simulink model "motor_dc_simulink"  (R2020a)
settings: Solver=VariableStepAuto  StartTime=0.0  StopTime=60  RelTol=1e-3
values from neighbouring files (symbols this model uses):
  b = 0    [Ex_AproximacaoDiscreta.m]    (also in Ex_PeriodoDeAmostragem1.m = 10; Ex_PeriodoDeAmostragem2.m = 17; motor_dc.m = 0.1)
  J = 0.01    [motor_dc.m]
  K = [0:0.001:30]    [Ex_LugarDasRaizes.m]    (also in Ex_ProjetoCtrlDireto.m = [0:0.005:50]; Ex_ProjetoCtrlDireto2.m = [0:0.001:50]; Ex_ProjetoCtrlEmulacao.m = [0:0.001:20]; Ex_ProjetoObsOrdemReduzida.m = [zeros(1,size(A,1)-1)  1]*inv(Co)*( A^2 + alphaccz(2)*A + al)
  L = [l1 l2]'    [Ex_ProjetoObservador.m]    (also in Ex_ProjetoObservador2.m = ( A^2 + alphacz(2)*A + alphacz(3)*eye(size(A)) )*inv(Ob)*[ze; Ex_ProjetoRastreamento.m = ( A^2 + alphacz(2)*A + alphacz(3)*eye(size(A)) )*inv(Ob)*[ze; motor_dc.m = 0.5)
  R = 1    [motor_dc.m]
  T = 0.1    [Ex_AproximacaoDiscreta.m]    (also in Ex_DiagramaDeBodeDiscreto.m = 1; Ex_LugarDasRaizes.m; Ex_PeriodoDeAmostragem1.m = 0.025; Ex_PeriodoDeAmostragem2.m = 0.0001)
undefined symbols (not defined in the file or in its folder): denaz_cl, numaz_cl, sigbuilder_block
libraries: simulink x1
settings Model: Creator=Dell  LastModifiedBy=Dell

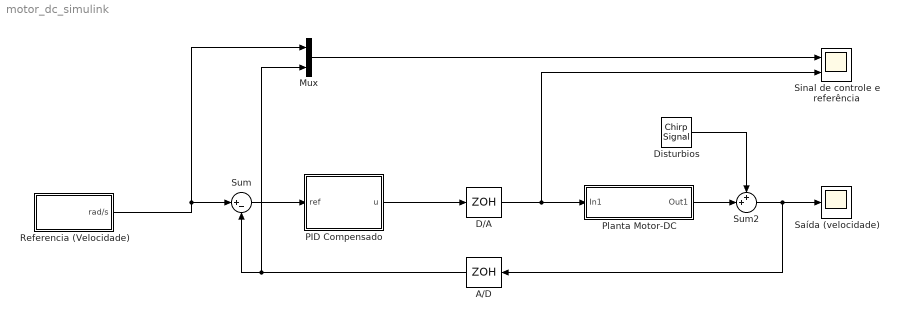
== system motor_dc_simulink ==
  A/D : ZeroOrderHold  SampleTime=T
  D/A : ZeroOrderHold  SampleTime=T
  Disturbios : simulink/Sources/Chirp Signal  f1=0.1  T=100  f2=1000
  Mux : Mux  Inputs=2
  PID Compensado : Subsystem
  Planta Motor-DC : Subsystem
  Referencia (Velocidade) : Subsystem  Tag=STV Subsys  LoadFcn=sigbuilder_block('load',[6 30 1012.5 447.75 ]);  StartFcn=sigbuilder_block('start');  StopFcn=sigbuilder_block('stop');  ClipboardFcn=sigbuilder_block('clipboard');  mask(Sigbuilder block){tuvar=[0:10]}
      mask help: Sigbuilder GUI
      mask init:
      | if ~strcmp(get_param(bdroot(gcbh),'SimulationStatus'),'stopped') tuvar = sigbuilder_block('maskInit'); end
      settings: CopyFcn=sigbuilder_block('copy');  DeleteFcn=sigbuilder_block('delete');  ModelCloseFcn=sigbuilder_block('modelClose');  PreSaveFcn=sigbuilder_block('preSave');  PauseFcn=sigbuilder_block('pause')  ContinueFcn=sigbuilder_block('continue')  NameChangeFcn=sigbuilder_block('namechange');  OpenFcn=sigbuilder_block('open',[6 30 1012.5 447.75 ]);  CloseFcn=sigbuilder_block('close');
      mask Display: plot(0, 0, 100, 100,[2, 2, 32, 32, 2], [68, 8, 8, 68, 68],[32, 2], [38, 38], [32, 19, 2],[53, 60, 44], [32, 17, 17, 2],[16, 16, 31, 31]);txt = getActiveGroup(gcbh);text(2, 100, txt,'verticalAlignment', 'top');
  Saída (velocidade) : Scope
  Sinal de controle e referência : Scope  NumInputPorts=2
  Sum : Sum  Inputs=|+-
  Sum2 : Sum  Inputs=++|
  wires:
  Sum/1 -> PID Compensado/1(ref)
  PID Compensado/1(u) -> D/A/1
  D/A/1 -> Planta Motor-DC/1(In1), Sinal de controle e referência/2
  Planta Motor-DC/1(Out1) -> Sum2/2
  Sum2/1 -> A/D/1, Saída (velocidade)/1
  A/D/1 -> Mux/2, Sum/2
  Mux/1 -> Sinal de controle e referência/1
  Referencia (Velocidade)/1(rad/s) -> Mux/1, Sum/1
  Disturbios/1 -> Sum2/1

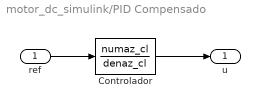
== system motor_dc_simulink/PID Compensado ==
  ref : Inport
  Controlador : DiscreteTransferFcn  Numerator=numaz_cl  Denominator=denaz_cl
  u : Outport
  wires:
  ref/1 -> Controlador/1
  Controlador/1 -> u/1

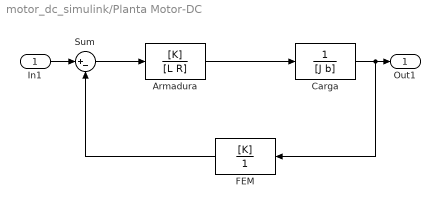
== system motor_dc_simulink/Planta Motor-DC ==
  In1 : Inport
  Armadura : TransferFcn  Numerator=[K]  Denominator=[L R]  ContinuousStateAttributes='torque'
  Carga : TransferFcn  Denominator=[J b]  ContinuousStateAttributes='velocidade'
  FEM : TransferFcn  Numerator=[K]  Denominator=1
  Sum : Sum  Inputs=|+-
  Out1 : Outport
  wires:
  In1/1 -> Sum/1
  Carga/1 -> FEM/1, Out1/1
  Armadura/1 -> Carga/1
  Sum/1 -> Armadura/1
  FEM/1 -> Sum/2

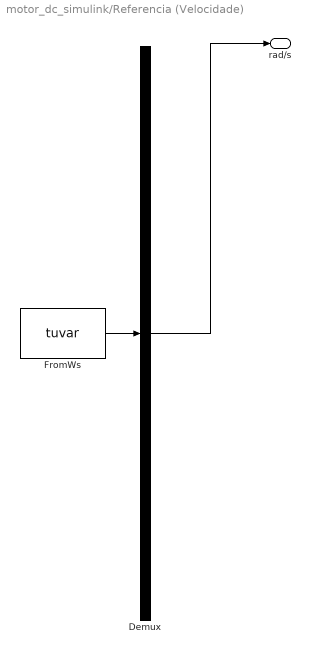
== system motor_dc_simulink/Referencia (Velocidade) ==
  Demux : Demux  Tag=STV Demux  Outputs=1
      settings: DisplayOption=none
  FromWs : FromWorkspace  Tag=STV FromWs  VariableName=tuvar
      SigBuilderData=|
      | common.afterFinalStr = 'Extrapolate'
      | common.sampleTime = 0
      | dataSet.timeRange = [0 60]
      | dataSet.name = 'Group 1'
      | sbobj.Groups.Name = 'Group 1'
      | sbobj.Groups.Signals.Name = 'rad/s'
      | sbobj.Groups.Signals.XData = [0 10 30 40 60]
      | sbobj.Groups.Signals.YData = [0 100 100 75 0]
      | sbobj.Groups.TimeRange = [0 60]
  rad/s : Outport  Tag=STV Outport
  wires:
  FromWs/1 -> Demux/1
  Demux/1 -> rad/s/1
